simulink model "c28069_lockedDC_T"  (R2018b)
settings: Solver=ode4  StartTime=0.0  StopTime=inf  FixedStep=Tsim  RelTol=1e-3
InitFcn:
  | %Ts=100e-6
  | Tsim = 0.0001
undefined symbols (not defined in the file or in its folder): serial
libraries: instrumentlib x2, powerlib_meascontrol x1
settings Model: Creator=matti  LastModifiedBy=matti
settings HardwareCC: ProdBitPerPointer=32  ProdBitPerSizeT=32  ProdBitPerPtrDiffT=32  ProdWordSize=32  ProdHWDeviceType=Intel->x86-32 (Windows32)
settings SFSimCC: SimUseLocalCustomCode=off
settings RTWCC: RTWUseLocalCustomCode=off
settings CodeAppCC: StateflowObjectComments=on
settings SimscapeCC: SimscapeNormalizeSystem=off

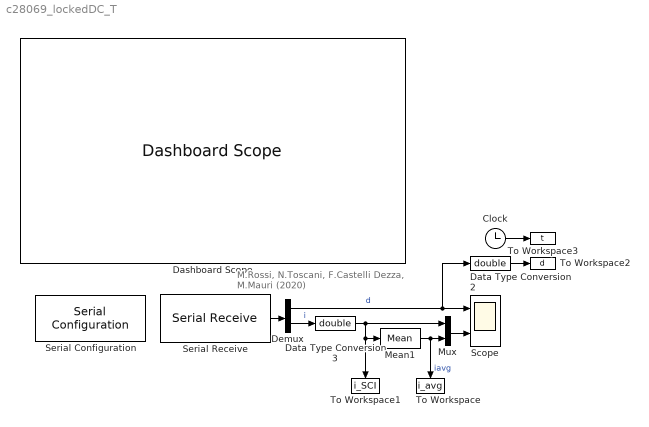
== system c28069_lockedDC_T ==
  note: M.Rossi, N.Toscani, F.Castelli Dezza, M.Mauri (2020)
  Clock : Clock
  Dashboard Scope : DashboardScope  WebBlockId=52  TimeSpan=100  Ymin=-0.10000000000000001  Ymax=1.1000000000000001
  Data Type Conversion2 : DataTypeConversion  OutDataTypeStr=double
  Data Type Conversion3 : DataTypeConversion  OutDataTypeStr=double
  Demux : Demux  Outputs=2
  Mean1 : powerlib_meascontrol/Measurements/Mean  Freq=50  Vinit=0  Ts=0
      settings: SourceProductName=Simscape Electrical
  Mux : Mux  Inputs=2
  Scope : Scope  NumInputPorts=2
  Serial Configuration : instrumentlib/Serial Configuration  Priority=-200000  ComPortMenu=<Please select a port...>  ComPort=COM14  ObjConstructor=serial('COM14');  BaudRate=115200  DataBits=8  Parity=none  StopBits=1  FlowControl=none  Timeout=10  ByteOrder=LittleEndian
  Serial Receive : instrumentlib/Serial Receive  ComPortMenu=<Please select a port...>  ComPort=<Please select a port...>  Terminator=<none>  DataSize="[1  2]"  DataType=single  EnableBlockingMode=on  ActionDataUnavailable=Output last received value  CustomValue=0  SampleTime=0.01
  To Workspace : ToWorkspace  VariableName=i_avg  SampleTime=0.0001
  To Workspace1 : ToWorkspace  VariableName=i_SCI  SampleTime=0.0001
      settings: Save2DSignal=2-D array (concatenate along first dimension)
  To Workspace2 : ToWorkspace  VariableName=d  SampleTime=0.0001
      settings: Save2DSignal=2-D array (concatenate along first dimension)
  To Workspace3 : ToWorkspace  VariableName=t  SampleTime=0.0001
      settings: Save2DSignal=2-D array (concatenate along first dimension)
  wires:
  Serial Receive/1 -> Demux/1
  Demux/1 -> Data Type Conversion2/1, Scope/1  "d"
  Demux/2 -> Data Type Conversion3/1  "i"
  Data Type Conversion2/1 -> To Workspace2/1
  Mean1/1 -> To Workspace/1, Mux/2  "iavg"
  Clock/1 -> To Workspace3/1
  Mux/1 -> Scope/2
  Data Type Conversion3/1 -> Mean1/1, To Workspace1/1, Mux/1
